simulink model "Obs_Avoi_with_sta_lin"  (R2023a)
settings: Solver=ode1  StartTime=0  StopTime=30  FixedStep=0.01  RelTol=1e-3
PostLoadFcn:
  | p=1:640; % pixels from left to right
  | 
  | Obtained_angles=(320-p).*(57/640)*pi./180;  % Kinect's horizontal FOV = 57 degrees
  | 
  | S=400; % S = Size of the 2D Map matrix... the highet S is the higher resolution we would end up with - %00 might be high for Embedded computing
values from neighbouring files (symbols this model uses):
  E = 0.3    [Main_Obst_Avoi_sta_lin.m]
  parameters = [R D omega Ts db  E b]    [Main_Obst_Avoi_sta_lin.m]
  Q0 = Qbd    [Main_Obst_Avoi_sta_lin.m]
  R = 0.035    [Main_Obst_Avoi_sta_lin.m]
  T = [R/2 R/2 ... (first row only)    [Main_Obst_Avoi_sta_lin.m]
  thetap = path.States(:,3)    [Main_Obst_Avoi_sta_lin.m]
  x = out.x.Data    [plots.m]
  X0 = p0    [Main_Obst_Avoi_sta_lin.m]
  xp = path.States(:,1)    [Main_Obst_Avoi_sta_lin.m]
  yp = path.States(:,2)    [Main_Obst_Avoi_sta_lin.m]
undefined symbols (not defined in the file or in its folder): gcbh, HIL, JPEG, qc_get_step_size, Video3D, video_display_show
libraries: quarc_library x29, simulink x3
(part 2 of 2)

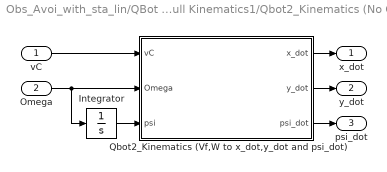
== system Obs_Avoi_with_sta_lin/QBot 2e Full Kinematics1/Qbot2_Kinematics (No Gyro) ==
  vC : Inport
  Omega : Inport  Port=2
  Integrator : Integrator
  Qbot2_Kinematics (Vf,W to x_dot,y_dot and psi_dot) : MATLAB Function  TreatAsAtomicUnit=on
  x_dot : Outport  VectorParamsAs1DForOutWhenUnconnected=off
  y_dot : Outport  Port=2  VectorParamsAs1DForOutWhenUnconnected=off
  psi_dot : Outport  Port=3  VectorParamsAs1DForOutWhenUnconnected=off
  wires:
  Qbot2_Kinematics (Vf,W to x_dot,y_dot and psi_dot)/3(psi_dot) -> psi_dot/1
  Integrator/1 -> Qbot2_Kinematics (Vf,W to x_dot,y_dot and psi_dot)/3(psi)
  vC/1 -> Qbot2_Kinematics (Vf,W to x_dot,y_dot and psi_dot)/1(vC)
  Qbot2_Kinematics (Vf,W to x_dot,y_dot and psi_dot)/1(x_dot) -> x_dot/1
  Omega/1 -> Integrator/1, Qbot2_Kinematics (Vf,W to x_dot,y_dot and psi_dot)/2(Omega)
  Qbot2_Kinematics (Vf,W to x_dot,y_dot and psi_dot)/2(y_dot) -> y_dot/1

== matlab function Obs_Avoi_with_sta_lin/MATLAB Function2 ==
  data: P_k_km1 input; P_kp1_k output; q input; u input; q_hat output; y input; Ts input
function [P_kp1_k,q_hat]= my_unscented_kalman_filter(P_k_km1,q,u,y,Ts)
Q=1e-6*eye(3);
R=1e-6*eye(3);
alpha=0.9; beta=2; kappa=0;
%Calculate the Sigma points
M=3;
c=alpha^2*(M+kappa);
q_hat_i=zeros(M,2*M+1);
q_hat_i(:,1)=q;
Delta_x=real(sqrtm(c*P_k_km1));
for i=1:M
    q_hat_i(:,i+1)=q+Delta_x(:,i);
    q_hat_i(:,i+1+M)=q-Delta_x(:,i);
end
%Output of the sigma points
y_hat_i=q_hat_i(1:3,:);
%predicted measurement at time k
W_M=zeros(1,2*M+1);
W_M(1)=1-(M/(alpha^2*(M+kappa)));
W_M(2:2*M+1)=(1/(2*alpha^2*(M+kappa)));
y_k=zeros(3,1);
for i=1:2*M+1
    y_k=y_k+W_M(i)*y_hat_i(:,i);
end
%Estimate of the covariance of predicted measurement
W_c=zeros(1,2*M+1);
W_c(1)=(2-alpha^2+beta)-(M/(alpha^2*(M+kappa)));
W_c(2:2*M+1)=(1/(2*alpha^2*(M+kappa)));
P_y=zeros(3,3);
for i=1:2*M+1
    P_y=P_y+W_c(i)*(y_hat_i(:,i)-y_k)*(y_hat_i(:,i)-y_k)'+R;
end
%%Estimate of the cross-covariance between predicted x and y
P_xy=zeros(M,3);
for i=1:2*M+1
    P_xy=P_xy+(1/(2*alpha^2*(M+kappa)))*(q_hat_i(:,i)-q)*(y_hat_i(:,i)-y_k)';
end
%Kalman gain
K=P_xy/(P_y);
q_k_k = q+K*(y-y_k);
P_k_k = P_k_km1 -K*P_y*K';
% State prediction and state estimation error covariance
q_hat_i_k_k=zeros(M,2*M+1);
q_hat_i_k_k(:,1)=q_k_k;
Delta_x=real(sqrtm(c*P_k_k));
for i=1:M
    q_hat_i_k_k(:,i+1)=q_k_k+Delta_x(:,i);
    q_hat_i_k_k(:,i+1+M)=q_k_k-Delta_x(:,i);
end
%Predicted state for each sigma point
q_hat_kp1_k=zeros(M,2*M+1);
for i=1:2*M+1
    q_hat_kp1_k(:,i)=q_hat_i_k_k(:,i)+Ts*[cos(q_hat_i_k_k(3,i)) 0;
        sin(q_hat_i_k_k(3,i)) 0;
        0          1]*u;
end
%Predicted state k+1 at time k
q_hat=zeros(M,1);
for i=1:2*M+1
    q_hat=q_hat + W_M(i)*q_hat_kp1_k(:,i);
end
%Covariance of the predicted state
P_kp1_k=zeros(M,M);
for i=1:2*M+1
    P_kp1_k=P_kp1_k+W_c(i)*(q_hat_kp1_k(:,i)-q_hat)*(q_hat_kp1_k(:,i)-q_hat)'+Q;
end
end

== matlab function Obs_Avoi_with_sta_lin/QBot 2e Inverse Kinematics (Forward Velocity and Angular Velocity into Left and Right Wheel Velocity)/Qbot2_Inverse_Kinematics (Forward Velocity and Angular Velocity into Left and Right Wheel Vellocity) ==
  data: vR output; vL output; vC input; Omega input
function [vR,vL] = fcn(vC , Omega)
%#codegen

d=0.235; 


vR = vC + Omega*d/2;
vL= vC - Omega*d/2;

== matlab function Obs_Avoi_with_sta_lin/MATLAB Function ==
  data: x input; Wr output; y input; theta input; Wl output; parameters input; Q0 input; wpx input; wpy input; wpt input
function [Wr, Wl] = fcn(x,y,theta, parameters, Q0, wpx,wpy,wpt)
%#codegen
coder.extrinsic("RHC_OA_stc_lin_mincx")
coder.extrinsic("dyn_FL_kothare_constraint_OA")
coder.extrinsic("RHC_OA_stc_lin")
R=parameters(1);        % radius od wheels [m]
D=parameters(2);        % distance between the two wheels [m]
omega=parameters(3);    % max angular velocity [rad/s] 
Ts=parameters(4);       % sampling time [s]
db=parameters(5);       % safe distance radius [m]
E=parameters(6);        % tolerance [m] 
b=parameters(7);        % distance point b [m]

u2=zeros(1,2)';

A=[1 0
    0 1];
B=[Ts 0
    0 Ts];
Hd=[-1/omega 0 1/omega 0;
    0 -1/omega 0 1/omega]';

T=[R/2 R/2;     % diff drive to unicycle
    R/D -R/D];
Tinv=inv(T);

Qbd=[db*db 0  % obstacle free ball shapping matrix 
    0 db*db];

Hu=Hd*Tinv;

Qe=eye(2);
rho=0.1;
Qu=rho*eye(2);

%Err = [x;y]-[wpx;wpy];
Err = [x+b*cos(theta);y+b*sin(theta)]-[wpx+b*cos(wpt);wpy+b*sin(wpt)];

Tflinv = [cos(theta) sin(theta);
          -sin(theta)/b cos(theta)/b];

H_theta = Hu*Tflinv;

%[Q_str,Y_str] = RHC_OA_stc_lin_mincx(Err,A,B,H_theta,Qbd,Qe,Qu);
%[Q_str,Y_str] = RHC_OA_stc_lin(Err,A,B,H_theta,Qbd,Qe,Qu);
 [Q_str,Y_str] =dyn_FL_kothare_constraint_OA(A,B,Err,Qe,Qu,H_theta,Q0);

u2 = Tinv*Tflinv*Y_str*inv(Q_str)*Err;


Wr=u2(1)*R;
Wl=u2(2)*R;

== matlab function Obs_Avoi_with_sta_lin/Reference trayectory ==
  data: Xr input; Yr input; thetap input; Xp input; Yp input; E input; k input; Wpx output; Wpy output; Wpt output; ypc input; xpc input; tpc input; k output; ypc output; xpc output; tpc output; err output
function [Wpx,Wpy,Wpt, k,ypc,xpc,tpc,err] = fcn(Xr,Yr,thetap, Xp,Yp, E, k,ypc,xpc,tpc)
coder.extrinsic("stopSimulation")
xp=double(Xp);
yp=double(Yp);
tp=double(thetap);
n_path=length(xp);
% persistent v1;
% persistent v2;
%     if isempty(v1)
%         v1 = 0;
%     end
%     if isempty(v2)
%         v2 = 0;
%     end
err=norm([Xr,Yr]-[xpc,ypc]);
if  norm([Xr,Yr]-[xpc,ypc])<=E
        if k<n_path
            k=k+1
            xpc=xp(k);
            ypc=yp(k);
            tpc=tp(k);
        elseif k==n_path
            xpc=xp(k);
            ypc=yp(k);
            tpc=tp(k);
            E=0.1;
            k=k+1
        else
           k=k+1
        end
end
Wpx=xpc;
Wpy=ypc;
Wpt=tpc;

== matlab function Obs_Avoi_with_sta_lin/Point Cloud ==
  data: D input; x output; y output; a input; psi input; d output
function [x, y, d]  = fcn(D,a,psi)
%#codegen


 psi = psi; 
 a = -a; 
  
    LINE=240;

    x=zeros(1,640);
    y=zeros(1,640);

    r=double(D(LINE,:))';
    %d=0.1236*tan((r/2842.5)+1.1863);
    d=r/1000;

    
    d(d<0.5) = 0;
    
%d((d<0.5)==1)=0;


    L=d./cos(a);

    x_r=L.*(cos(-a));
    y_r=L.*(sin(-a));
        

   
    
    R=[cos(psi) -sin(psi)
    sin(psi) cos(psi)];

   
    for j=1:640
        XY=R*[x_r(j);y_r(j)];
        x(j)=XY(1);
        y(j)=XY(2);
    end

    
  %alpha= -(LINE-240)*43*pi/180/480; % Vertical FOV
  %z=  tan(alpha)*L.*ones(640,1);

== matlab function Obs_Avoi_with_sta_lin/Motion Planning and Control ==
  settings: sampleTime=qc_get_step_size
  data: x input; y input; theta input; Vc output; Omega output; flags output; ENABLE output
function [Vc, Omega, flags, ENABLE] = fcn(x,y,theta)
%#codegen


persistent v;
persistent w;
persistent flag_rotate
persistent flag_move
persistent flag_rotate_back
persistent flag_move_back
persistent enable;
persistent EN;


if isempty(flag_rotate)
    flag_rotate=0;
end

if isempty(flag_move)
    flag_move=0;
end

if isempty(flag_rotate_back)
    flag_rotate_back=0;
end

if isempty(flag_move_back)
    flag_move_back=0;
end

if isempty(v)
    v=0;
end

if isempty(w)
    w=0;
end

if isempty(enable)
    enable=1;
end

if isempty(EN)
    EN=1;
end

%if buttons==1
%    EN=1;
%elseif buttons==2
%    enable=1;
%elseif buttons==4
%    enable=0;
%end


%if bumpers~=1 && bumpers~=2 && bumpers~=4 && bumpers~=3 && bumpers~=5 && bumpers~=6
    if flag_rotate==0 && theta<2*pi-0.05
       % w=0.25;
         w=0.3*(2*pi-theta);
         v=0;
    elseif flag_rotate==0 && theta>2*pi-0.05 && theta<2*pi+0.05
        flag_rotate=1;
    %    w=0;
    %    v=0;
    end

    if flag_rotate==1 && flag_move==0 && x<0.5;
        w=0;
        v=0.2;
    elseif flag_rotate==1 && flag_move==0 &&  x>0.45 && x<0.55
        flag_move=1;
        w=0;
        v=0;
    end


    if flag_move==1 && flag_rotate_back==0 && theta>pi+0.05 
        %w=-0.25;
        w=0.3*(pi-theta);
        v=0;
    elseif flag_move==1 && flag_rotate_back==0 && theta<pi+0.05  && theta>pi-0.05
        flag_rotate_back=1;
 %       w=0;
 %       v=0;
    end

    if flag_rotate_back==1 && flag_move_back==0 && x>0.05;
%        w=0.1*(pi-theta);
        v=0.2;
    elseif flag_rotate_back==1 && flag_move_back==0 &&  x<0.05 && x>-0.05
        flag_move_back=1;
        w=0;
        v=0;
    end    
%else
%    enable=0;
%     w=0;
%     v=0;
%end
    
if abs(w)>0.4 
       w=sign(w)*0.4;
end
            
if abs(v)>0.3 
       v=sign(v)*0.25;
end


flags=[flag_rotate, flag_move, flag_rotate_back, flag_move_back];
        
Vc=v*enable;
Omega=w*enable;
ENABLE=EN;

== matlab function Obs_Avoi_with_sta_lin/QBot 2e Full Kinematics/Qbot2_Diff_Drive_Kinematics/Qbot2_Diff_Drive_Kinematics ==
  data: vL input; vC output; vR input; Omega output
function [vC,Omega] = fcn(vL,vR)
%#codegen

d= 0.235;

vC=0.5*(vL+vR);
Omega=(1/d)*(vR-vL);

== matlab function Obs_Avoi_with_sta_lin/QBot 2e Full Kinematics/Qbot2_Kinematics (No Gyro)/Qbot2_Kinematics (Vf,W to x_dot,y_dot and psi_dot) ==
  data: vC input; x_dot output; Omega input; y_dot output; psi input; psi_dot output
function [x_dot,y_dot,psi_dot] = fcn(vC,Omega,psi)
%#codegen


x_dot=cos(psi)*vC;
y_dot=sin(psi)*vC;
psi_dot= Omega;

== matlab function Obs_Avoi_with_sta_lin/2D Map Update ==
  settings: sampleTime=qc_get_step_size
  data: x_cin input; y_cin input; xin input; yin input; y1 output
function y1 = fcn(x_cin,y_cin,xin, yin)
%#codegen

S=100;
scale=S/20;

x = round(xin*scale);
y = round(yin*scale);

x_c = round(x_cin*scale+x);
y_c = round(y_cin*scale+y);

%z_c = round(x_c*scale+0);

persistent M;

if isempty(M)
    M=uint8(100*ones(S+1,S+1));
end



    for i=1:length(x_c)

         M((x_c(i)+S/2+1),(y_c(i)+S/2+1))=0; % matrix indices start from 1 + centre the data


        
        % refreshing the old data within the FOV cone
        Dist_Lx= (x_c(i)-x);
        Dist_Ly=(y_c(i)-y);
        L=[Dist_Lx,Dist_Ly];


        [m, m_idx] = max([abs(L(1)), abs(L(2))]);

        if m>0
            if m_idx(1)==1 % diff in x is larger
                for k=0: sign(L(1)): x_c(i)-x - sign(L(1))
                    M(x+S/2+k+1,y+round(Dist_Ly*k/Dist_Lx)+S/2+1)=255;
                end
            end

            if m_idx(1)==2
                for k=0: sign(L(2)): y_c(i)-y - sign(L(2))
                    M(x+round(Dist_Lx*k/Dist_Ly)+S/2+1,y+k+S/2+1)=255;
                end
            end
        end
         
        


    end



y1=M;

== matlab function Obs_Avoi_with_sta_lin/QBot 2e Full Kinematics1/Qbot2_Diff_Drive_Kinematics/Qbot2_Diff_Drive_Kinematics ==
  data: vL input; vC output; vR input; Omega output
function [vC,Omega] = fcn(vL,vR)
%#codegen

d= 0.235;

vC=0.5*(vL+vR);
Omega=(1/d)*(vR-vL);

== matlab function Obs_Avoi_with_sta_lin/QBot 2e Full Kinematics1/Qbot2_Kinematics (No Gyro)/Qbot2_Kinematics (Vf,W to x_dot,y_dot and psi_dot) ==
  data: vC input; x_dot output; Omega input; y_dot output; psi input; psi_dot output
function [x_dot,y_dot,psi_dot] = fcn(vC,Omega,psi)
%#codegen


x_dot=cos(psi)*vC;
y_dot=sin(psi)*vC;
psi_dot= Omega;
